simulink model "model_v1"  (R2018b)
settings: Solver=VariableStepAuto  StartTime=0.0  StopTime=10.0  RelTol=1e-3
settings Model: Creator=rarora  LastModifiedBy=rarora

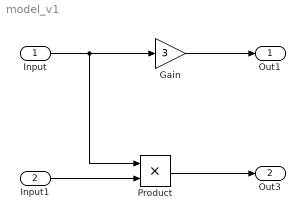
== system model_v1 ==
  Input : Inport
  Input1 : Inport  Port=2
  Gain : Gain  Gain=3
  Product : Product
  Out1 : Outport
  Out3 : Outport  Port=2
  wires:
  Product/1 -> Out3/1
  Input1/1 -> Product/2
  Input/1 -> Product/1, Gain/1
  Gain/1 -> Out1/1
